simulink model "mmsimplerobot_test"  (R2025a)
settings: Solver=VariableStepAuto  StartTime=0.0  StopTime=10.0  RelTol=1e-3
undefined symbols (not defined in the file): simstruct
libraries: mmuct_lib x6, dhaouadi2013_lib x2
settings Model: Creator=nicolls  LastModifiedBy=sanjannaidoo

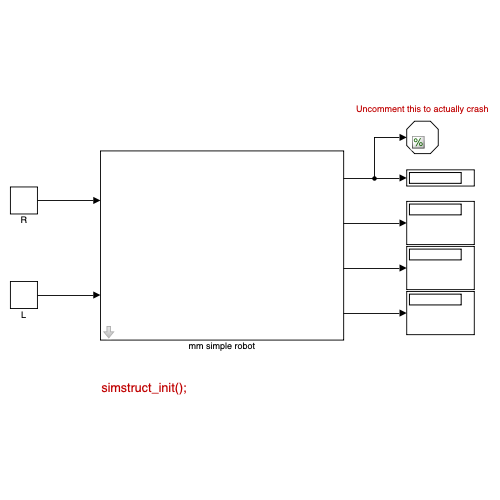
[thumbnail: Simulink's stored preview of the top-level diagram]
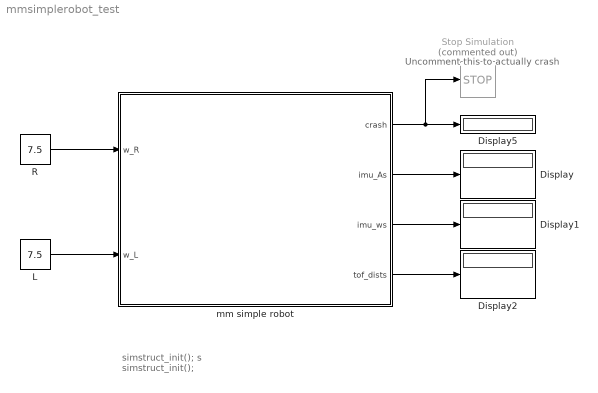
== system mmsimplerobot_test ==
  note: Uncomment this to actually crash
  note: simstruct_init();
      | s
      | simstruct_init();
  Display{,1..2,5} (4 alike) : Display
  L : Constant  Value=7.5
  R : Constant  Value=7.5
  Stop Simulation : Stop  Commented=on
  mm simple robot : Subsystem  mask{simstruct=simstruct}
      mask prompts: simstruct "Simulation structure variable"
      mask Display: image('uctmm_image.png');
  wires:
  L/1 -> mm simple robot/2(w_L)
  R/1 -> mm simple robot/1(w_R)
  mm simple robot/1(crash) -> Stop Simulation/1, Display5/1
  mm simple robot/2(imu_As) -> Display/1
  mm simple robot/3(imu_ws) -> Display1/1
  mm simple robot/4(tof_dists) -> Display2/1

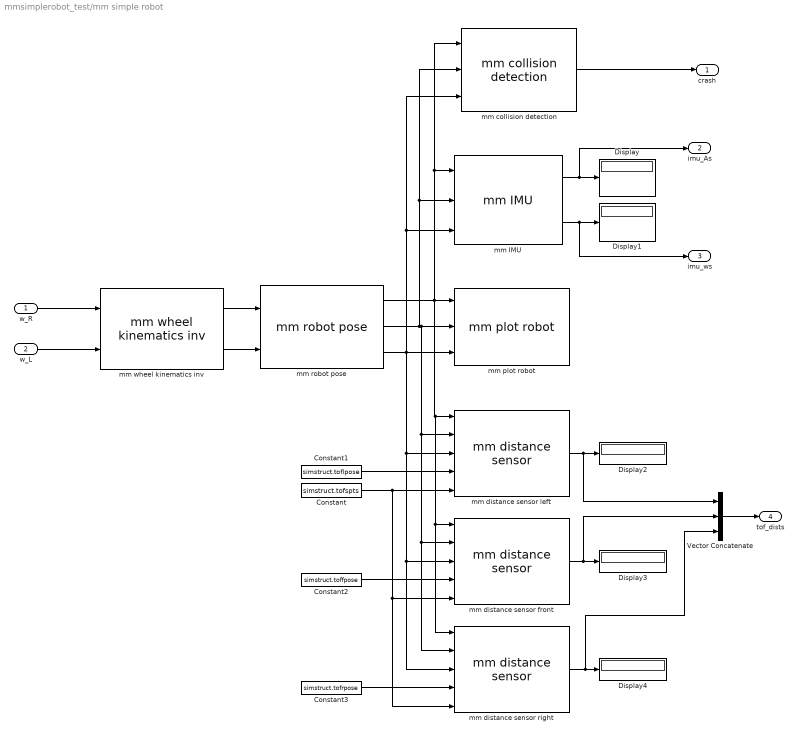
== system mmsimplerobot_test/mm simple robot ==
  w_R : Inport
  w_L : Inport  Port=2
  Constant : Constant  Value=simstruct.tofspts
  Constant1 : Constant  Value=simstruct.toflpose
  Constant2 : Constant  Value=simstruct.toffpose
  Constant3 : Constant  Value=simstruct.tofrpose
  Display{,1..4} (5 alike) : Display
  Vector Concatenate : Concatenate  NumInputs=3
  mm IMU : mmuct_lib/mm IMU  SystemSampleTime=-1  VariantActivationTime=update diagram  EmptyChoice=off  PassThrough=off  PassThroughVariantControl=(default)  EmptyChoiceVariantControl=(default)  AllowFlexibleInterface=on  Latency=0  AutoFrameSizeCalculation=off
      settings: SourceProductName=UCT EEE Micromouse
  mm collision detection : mmuct_lib/mm collision detection  simstruct=simstruct
      settings: SourceProductName=UCT EEE Micromouse
  mm distance sensor front : mmuct_lib/mm distance sensor  simstruct=simstruct  debug=0
  mm distance sensor left : mmuct_lib/mm distance sensor  simstruct=simstruct  debug=0
      settings: SourceProductName=UCT EEE Micromouse
  mm distance sensor right : mmuct_lib/mm distance sensor  simstruct=simstruct  debug=0
      settings: SourceProductName=UCT EEE Micromouse
  mm plot robot : mmuct_lib/mm plot robot  x0=0.1  y0=0.1  theta0=0  simstruct=simstruct
      settings: SourceProductName=UCT EEE Micromouse
  mm robot pose : dhaouadi2013_lib/mm robot pose  x0=0.1  y0=0.1  theta0=0
  mm wheel kinematics inv : dhaouadi2013_lib/mm wheel kinematics inv  L=simstruct.L  R=simstruct.R
  crash : Outport
  imu_As : Outport  Port=2
  imu_ws : Outport  Port=3
  tof_dists : Outport  Port=4
  wires:
  Constant/1 -> mm distance sensor right/5, mm distance sensor front/5, mm distance sensor left/5
  mm distance sensor front/1 -> Vector Concatenate/2, Display3/1
  mm wheel kinematics inv/2 -> mm robot pose/2
  Constant2/1 -> mm distance sensor front/4
  Constant1/1 -> mm distance sensor left/4
  mm robot pose/2 -> mm distance sensor right/2, mm distance sensor front/2, mm distance sensor left/2, mm plot robot/2, mm collision detection/2, mm IMU/2
  Constant3/1 -> mm distance sensor right/4
  mm IMU/2 -> imu_ws/1, Display1/1
  mm IMU/1 -> imu_As/1, Display/1
  mm wheel kinematics inv/1 -> mm robot pose/1
  mm robot pose/1 -> mm IMU/1, mm collision detection/1, mm distance sensor right/1, mm distance sensor front/1, mm distance sensor left/1, mm plot robot/1
  mm distance sensor right/1 -> Vector Concatenate/3, Display4/1
  mm robot pose/3 -> mm collision detection/3, mm IMU/3, mm distance sensor right/3, mm distance sensor front/3, mm distance sensor left/3, mm plot robot/3
  mm collision detection/1 -> crash/1
  mm distance sensor left/1 -> Vector Concatenate/1, Display2/1
  Vector Concatenate/1 -> tof_dists/1
  w_L/1 -> mm wheel kinematics inv/2
  w_R/1 -> mm wheel kinematics inv/1
